simulink model "mqam_2020a"  (R2020a)
settings: Solver=VariableStepAuto  StartTime=0.0  StopTime=10.0  RelTol=1e-3
PreLoadFcn:
  | %%% model parameters %%%
  | 
  | Rb = 10e6; % bit rate
  | Tb = 1/Rb; % bit interval
  | 
  | M = 256; % constelation alphabet
  | Nb = log2(M); % number of bit
  | 
  | Rs = Rb/Nb; % symbol rate
  | N = 100; % number of samples per symbol
  | R = N*Rs; % sampling rate
  | 
  | fc = 100e6; % carrier frequency
  | 
  | Eg = 1 %
  | 
  | 
  | %%% gray code mapper %%%
  | 
  | gray_codes = get_gray_codes(Nb/2);
  | 
  | gray_cont = containers.Map % container
  | for i=1:size(gray_codes,2)
  |   binary_str = num2str(flip(gray_codes(:,i)'));
  |   binary_str(binary_str == ' ') = '';
  |   gray_cont(binary_str) = (i-1)*2 - ((M/4 -1)*2 + 1);
  | end
InitFcn:
  | phi = 0; % phase offset
undefined symbols (not defined in the file or in its folder): fdesignblkfcn, gcbh, magnitude
libraries: dspstat3 x3, dspsrcs4 x3, commchan3 x1, commfilt2 x1, commrandsrc3 x1, dsparch4 x1, commsink2 x1
settings Model: Creator=tapyu  LastModifiedBy=tapyu
settings DebuggingCC: UnconnectedInputMsg=none  UnconnectedOutputMsg=none  UnconnectedLineMsg=none  SFMachineParentedDataDiag=error

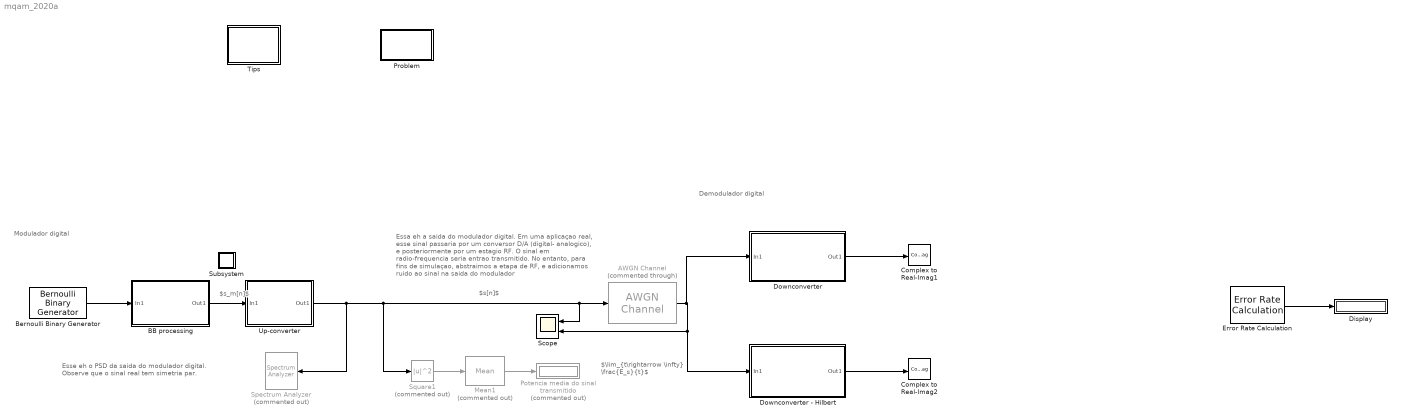
== system mqam_2020a ==
  note: Demodulador digital
  note: Essa eh a saida do modulador digital. Em uma aplicaçao
      | real, esse sinal passaria por um conversor D/A (digital-
      | analogico), e posteriormente por um estagio RF. O sinal
      | em radio-frequencia seria entrao transmitido. No entanto,
      | para fins de simulaçao, abstraimos a etapa de RF,
      | e adicionamos ruido ao sinal na saida do modulador
  note: $s[n]$
  note: Esse eh o PSD da saida do modulador digital.
      | Observe que o sinal real tem simetria par.
  note: Modulador digital
  note: $s_m[n]$
  note: $\lim_{t\rightarrow \infty} \frac{E_s}{t}$
  AWGN Channel : commchan3/AWGN Channel  Commented=through  InputProcessing=Columns as channels (frame based)  seed=67  noiseMode="Signal to noise ratio  (Eb/No)"  EbNodB=10  EsNodB=10  SNRdB=10  bitsPerSym=sqrt(M)  Ps=1  Tsym=Tb  variance=1
  BB processing : Subsystem
  Bernoulli Binary Generator : commrandsrc3/Bernoulli Binary Generator  ProbabilityOfZero=0.5  SeedSource=Auto  Seed=0  SampleTime=Tb  SamplesPerFrame=1  OutputDataType=double  SimulateUsing=Interpreted execution
  Complex to Real-Imag1 : ComplexToRealImag
  Complex to Real-Imag2 : ComplexToRealImag
  Display : Display
  Downconverter : Subsystem
  Downconverter - Hilbert : Subsystem
  Error Rate Calculation : commsink2/Error Rate Calculation  N=0  st_delay=0  cp_mode=Entire frame  subframe=[]  PMode=Port  WsName=ErrorVec  RsMode2=off  stop=off  numErr=100  maxBits=1e6
  Mean1 : dspstat3/Mean  Commented=on  run=on  reset_popup=None  directionMode=Entire input  dimension=1  roiEnable=off  roiType=Rectangles  roiPortion=Entire ROI  roiOutput=Individual statistics for each ROI  roiFlag=off  roundingMode=Floor  overflowMode=off  outputDataTypeStr=Inherit: Same as accumulator  outputMin=[]  outputMax=[]  outputLastDataTypeStr=Inherit: Same as accumulator
  Potencia media do sinal transmitido : Display  Commented=on
  Problem : Subsystem
  Scope : Scope  NumInputPorts=2
  Spectrum Analyzer : SpectrumAnalyzer  Commented=on
  Square1 : Math  Commented=on  Operator=magnitude^2  SaturateOnIntegerOverflow=on
  Subsystem : Subsystem
  Tips : Subsystem
  Up-converter : Subsystem
  wires:
  BB processing/1(Out1) -> Up-converter/1(In1)
  Up-converter/1(Out1) -> Spectrum Analyzer/1, Square1/1, Scope/1, AWGN Channel/1
  Mean1/1 -> Potencia media do sinal transmitido/1
  Square1/1 -> Mean1/1
  AWGN Channel/1 -> Downconverter/1(In1), Downconverter - Hilbert/1(In1), Scope/2
  Bernoulli Binary Generator/1 -> BB processing/1(In1)
  Error Rate Calculation/1 -> Display/1
  Downconverter/1(Out1) -> Complex to Real-Imag1/1
  Downconverter - Hilbert/1(Out1) -> Complex to Real-Imag2/1

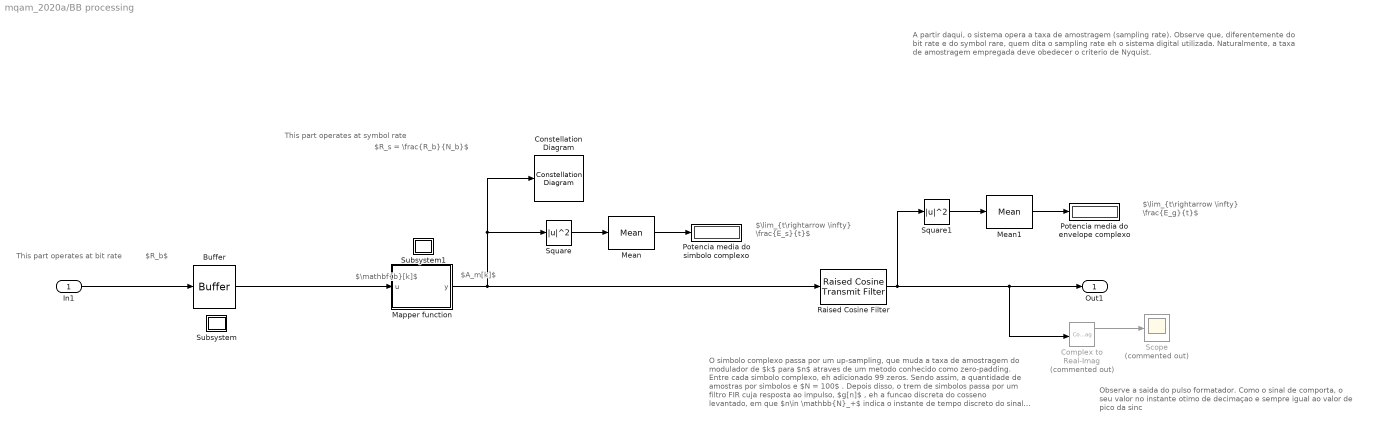
== system mqam_2020a/BB processing ==
  note: A partir daqui, o sistema opera a taxa de amostragem (sampling rate).
      | Observe que, diferentemente do bit rate e do symbol rare, quem dita o sampling rate
      | eh o sistema digital utilizada. Naturalmente, a taxa de amostragem empregada deve
      | obedecer o criterio de Nyquist.
  note: Observe a saida do pulso formatador. Como o sinal de comporta,
      | o seu valor no instante otimo de decimaçao e sempre igual ao
      | valor de pico da sinc
  note: $\lim_{t\rightarrow \infty} \frac{E_s}{t}$
  note: $R_s = \frac{R_b}{N_b}$
  note: This part operates
      | at symbol rate
  note: $R_b$
  note: This part operates at bit rate
  note: O simbolo complexo passa por um up-sampling, que muda a taxa de amostragem do modulador de $k$ para $n$ atraves de um metodo conhecido como zero-padding. Entre cada simbolo complexo, eh adicionado 99 zeros. Sendo assim, a quantidade de amostras por simbolos e $N = 100$ . Depois disso, o trem de simbolos passa por um filtro FIR cuja resposta ao impulso, $g[n]$ , eh a funcao discreta do cosseno levantado, em que $n\in \mathbb{N}_+$ indica o instante de tempo discreto do sinal que opera a taxa de amostragem, $R=N R_s$ . O sinal de saida do filtro para o k-esimo simbolo transmitido eh dado por $s[n] = A_m[k] g[n]$ . Este sinal eh comumente referido como envelope complexo. Clique no bloco do filtro cosseno levantado->view filter response e observe os seguintes pontos:
      |
      | - Resposta ao impulso do filtro cosseno levantado eh na verdade uma versao truncada da mesma em 4 intervalos de simbolos (recorde que cada intervalo de simbolos contem $N = 100$ amostras). O motivo disso eh a factibilidade na hora da implementaçao: nao eh possivel definir um filtro FIR com resposta ao impulso de duraçao infinita, por isso faz-se necessario trunca-la. Observe que o efeito to truncamento no tempo leva a uma distorçao da resposta em frequencia do filtro FIR. Tem-se entao um termo de compromisso (trade-off) entre o tramanho da janela de truncamento e nivel de distorçao da resposta de frequencia.
      |
      | - Oberseve que, embora haja sobreposiçao entre os simbolos vizinhos, ha interferencia nula nos instantes otimos de decimaçao: conte $100$ amostras a partir do instante de pico e vera que pulso cruza o valor zero nesses instantes. Isso ocorre porque o pulso cosseno levantado respeita o criterio de Nyquist de nao ISI.
      |
      | - A amplitude do cosseno levantado eh modificada de tal forma que $E_g = 1$$
  note: $A_m[k]$
  note: $\mathbf{b}[k]$
  note: $\lim_{t\rightarrow \infty} \frac{E_g}{t}$
  In1 : Inport
  Buffer : Buffer  N=Nb  OutputFrames=off
  Complex to Real-Imag : ComplexToRealImag  Commented=on
  Constellation Diagram : ConstellationDiagram
  Mapper function : MATLAB Function  TreatAsAtomicUnit=on
  Mean : dspstat3/Mean  run=on  reset_popup=None  directionMode=Entire input  dimension=1  roiEnable=off  roiType=Rectangles  roiPortion=Entire ROI  roiOutput=Individual statistics for each ROI  roiFlag=off  roundingMode=Floor  overflowMode=off  outputDataTypeStr=Inherit: Same as accumulator  outputMin=[]  outputMax=[]  outputLastDataTypeStr=Inherit: Same as accumulator
  Mean1 : dspstat3/Mean  run=on  reset_popup=None  directionMode=Entire input  dimension=1  roiEnable=off  roiType=Rectangles  roiPortion=Entire ROI  roiOutput=Individual statistics for each ROI  roiFlag=off  roundingMode=Floor  overflowMode=off  outputDataTypeStr=Inherit: Same as accumulator  outputMin=[]  outputMax=[]  outputLastDataTypeStr=Inherit: Same as accumulator
  Potencia media do envelope complexo : Display
  Potencia media do simbolo complexo : Display
  Raised Cosine Filter : commfilt2/Raised Cosine Transmit Filter  filtType=Normal  R=0.2  filtSpan=4  N=N  filterGain=sqrt(N)  RateOptions=Allow multirate processing  framing=Mute  checkCoeff=off  variableName=rcTxFilt  checkGain=Normalized  sampMode=Mute  saveAsFlag=0  currentFiltSpan=4  D=(4)/2  launchFVT=on  roundingMode=Floor  overflowMode=off  coeffDataTypeStr=Inherit: Same word length as input  coeffMin=[]  coeffMax=[]  coeffLastDataTypeStr=Inherit: Same word length as input  outputDataTypeStr=Inherit: Same as accumulator  outputMin=[]  outputMax=[]  outputLastDataTypeStr=Inherit: Same as accumulator
  Scope : Scope  Commented=on
  Square : Math  Operator=magnitude^2  SaturateOnIntegerOverflow=on
  Square1 : Math  Operator=magnitude^2  SaturateOnIntegerOverflow=on
  Subsystem : Subsystem
  Subsystem1 : Subsystem
  Out1 : Outport
  wires:
  Buffer/1 -> Mapper function/1(u)
  Mean/1 -> Potencia media do simbolo complexo/1
  Mapper function/1(y) -> Constellation Diagram/1, Square/1, Raised Cosine Filter/1
  Square/1 -> Mean/1
  In1/1 -> Buffer/1
  Mean1/1 -> Potencia media do envelope complexo/1
  Square1/1 -> Mean1/1
  Complex to Real-Imag/1 -> Scope/1
  Raised Cosine Filter/1 -> Complex to Real-Imag/1, Out1/1, Square1/1

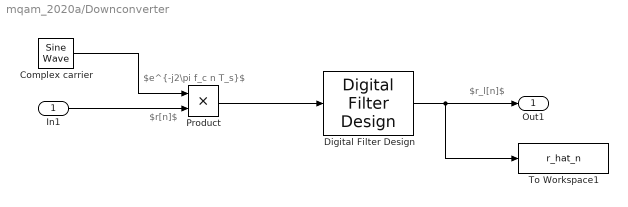
== system mqam_2020a/Downconverter ==
  note: $r[n]$
  note: $e^{-j2\pi f_c n T_s}$
  note: $r_l[n]$
  In1 : Inport
  Complex carrier : dspsrcs4/Sine Wave  Amplitude=sqrt(2/Eg)  Frequency=fc  Phase=0  SampleMode=Discrete  OutComplex=Complex  CompMethod=Trigonometric fcn  TableSize=Speed  SampleTime=1/R  SamplesPerFrame=1  ResetState=Restart at time zero  OutputFrames=off  dataType=double  wordLen=16  udDataType=sfix(16)  fracBitsMode=Best precision  numFracBits=15  OutDataTypeStr=double  LastOutDataTypeStr=double
  Digital Filter Design : dsparch4/Digital Filter Design  mwdsp_browser_bugfix_var=off
  Product : Product
  To Workspace1 : ToWorkspace  VariableName=r_hat_n  SaveFormat=Timeseries  SampleTime=-1
  Out1 : Outport
  wires:
  In1/1 -> Product/2
  Complex carrier/1 -> Product/1
  Product/1 -> Digital Filter Design/1
  Digital Filter Design/1 -> To Workspace1/1, Out1/1

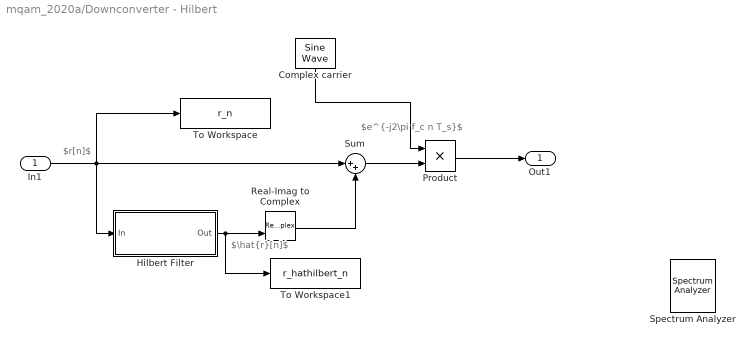
== system mqam_2020a/Downconverter - Hilbert ==
  note: $e^{-j2\pi f_c n T_s}$
  note: $r[n]$
  note: $\hat{r}[n]$
  In1 : Inport
  Complex carrier : dspsrcs4/Sine Wave  Amplitude=sqrt(2/Eg)  Frequency=-fc  Phase=0  SampleMode=Discrete  OutComplex=Complex  CompMethod=Trigonometric fcn  TableSize=Speed  SampleTime=1/R  SamplesPerFrame=1  ResetState=Restart at time zero  OutputFrames=off  dataType=double  wordLen=16  udDataType=sfix(16)  fracBitsMode=Best precision  numFracBits=15  OutDataTypeStr=double  LastOutDataTypeStr=double
  Hilbert Filter : Subsystem  DialogController=fdesignblkfcn  InitFcn=fdesignblkfcn(gcbh, {'InitFcn'});  mask(Hilbert Filter){}
      mask help: Design a Hilbert filter
      settings: CopyFcn=fdesignblkfcn(gcbh, {'CopyFcn'});
      mask Help: helpview(mapfilelocation('dsp'), 'dsphilbertfilter');
      mask Display: disp('Hilbert')
  Product : Product
  Real-Imag to Complex : RealImagToComplex
  Spectrum Analyzer : SpectrumAnalyzer  NumInputPorts=2
  Sum : Sum  Inputs=|++
  To Workspace : ToWorkspace  VariableName=r_n  SaveFormat=Timeseries  SampleTime=-1
  To Workspace1 : ToWorkspace  VariableName=r_hathilbert_n  SaveFormat=Timeseries  SampleTime=-1
  Out1 : Outport
  wires:
  Sum/1 -> Product/2
  Complex carrier/1 -> Product/1
  Product/1 -> Out1/1
  In1/1 -> Sum/1, To Workspace/1, Hilbert Filter/1(In)
  Hilbert Filter/1(Out) -> To Workspace1/1, Real-Imag to Complex/2
  Real-Imag to Complex/1 -> Sum/2

== system mqam_2020a/Problem ==
  note: Bit rate:

== system mqam_2020a/Subsystem ==
  note: This is the complex envelope, also called the low-pass equivalent of the modulation scheme.

== system mqam_2020a/Tips ==
  note: Tips:
      |
      | - Go to debug->information overlays to set/unset visual indicators (called overlays). The main ones are: colors, timing legend, signals dimensions, base data types
      | - Go to modeling->model explorer->mqam->callbacks->PreLoadFnc to see the variables declared in this Simulink model. They are visible in the workspace area of the main window. In addition they can also be changed in the command window.

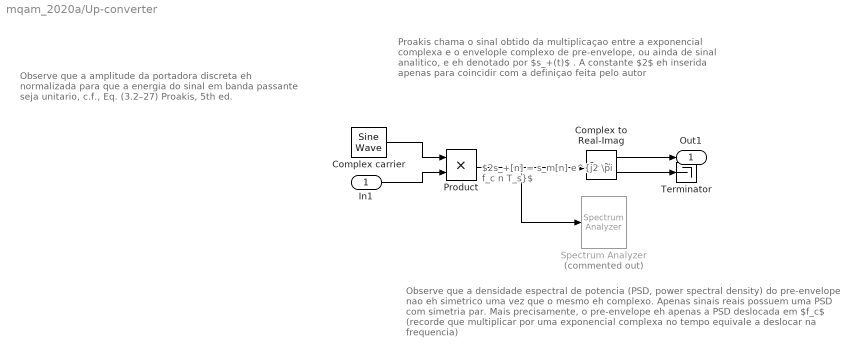
== system mqam_2020a/Up-converter ==
  note: Observe que a amplitude da portadora discreta eh
      | normalizada para que a energia do sinal em banda
      | passante seja unitario, c.f., Eq. (3.2–27) Proakis, 5th ed.
  note: Observe que a densidade espectral de potencia (PSD, power spectral density) do pre-envelope nao eh simetrico uma vez que o mesmo eh complexo.
      | Apenas sinais reais possuem uma PSD com simetria par. Mais precisamente, o pre-envelope eh apenas a PSD deslocada em $f_c$ (recorde que multiplicar por uma exponencial complexa no tempo equivale a deslocar na frequencia)
  note: Proakis chama o sinal obtido da multiplicaçao entre a exponencial
      | complexa e o envelople complexo de pre-envelope, ou ainda de
      | sinal analitico, e eh denotado por $s_+(t)$ . A constante $2$ eh inserida
      | apenas para coincidir com a definiçao feita pelo autor
  note: $2s_+[n] = s_m[n] e^{j2 \pi f_c n T_s}$
  In1 : Inport
  Complex carrier : dspsrcs4/Sine Wave  Amplitude=sqrt(2)  Frequency=fc  Phase=0  SampleMode=Discrete  OutComplex=Complex  CompMethod=Trigonometric fcn  TableSize=Speed  SampleTime=1/R  SamplesPerFrame=1  ResetState=Restart at time zero  OutputFrames=off  dataType=double  wordLen=16  udDataType=sfix(16)  fracBitsMode=Best precision  numFracBits=15  OutDataTypeStr=double  LastOutDataTypeStr=double
  Complex to Real-Imag : ComplexToRealImag
  Product : Product
  Spectrum Analyzer : SpectrumAnalyzer  Commented=on
  Terminator : Terminator
  Out1 : Outport
  wires:
  Complex carrier/1 -> Product/1
  In1/1 -> Product/2
  Complex to Real-Imag/1 -> Out1/1
  Product/1 -> Spectrum Analyzer/1, Complex to Real-Imag/1
  Complex to Real-Imag/2 -> Terminator/1

== system mqam_2020a/BB processing/Subsystem ==
  note: The bitstream operates at a rate of $R_b = 10 Mbps$ . The first task is to transform the stream bit into a vector, $\mathbf{b}[k] \in \mathbb{R}^{K}$ , where $k \in \mathbb{N}_+$ is the $k$ th set of $K = \log_2 (M)$ bits

== system mqam_2020a/BB processing/Subsystem1 ==
  note: Each sequence of $K = \log_2(M)$ bit is mapped (using Gray code) to a complex symbol, $A_m[k]$ , where $m \in \{1,2,\cdots,M\}$ is the $m$ th complex symbol of the alphabet, and $k \in \mathbb{N}_+$ is the $k$ th transmitted symbol

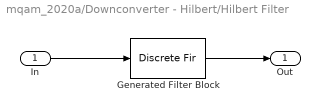
== system mqam_2020a/Downconverter - Hilbert/Hilbert Filter ==
  In : Inport
  Generated Filter Block : DiscreteFir  Tag=BlockMethodSubSystem  Coefficients=[-0.379139248397066475 -6.14990643046237073e-15 -0.0322139499300219123 -1.08779359218186267e-15 -0.0337279953162739066 -1.6870185803874449e-15 -0.0362439670869629804 -2.70443389904784226e-15 -0.0398003827467814375 5.01855501600090292e-15 -0.0445494339270779971 -2.66236685475540469e-15 -0.0508633445439188314 5.47305256670682638e-16 -0.0595171048736182762 -1.85441939581920678e-15 -0.0720795865005312564 7.71951946809679157e-16 -0.0919627441700265891 -6.38378239159465011e-16 -0.128017407479324774 1.11022302462515654e-16 -0.212602811441472639 -3.26128013483639734e-16 -0.636747756767987561 0 0.636747756767987561 3.26128013483639734e-16 0.212602811441472639 -1.11022302462515654e-16 0.128017407479324774 6.38378239159465011e-16 0.0919627441700265891 -7.71951946809679157e-16 0.0720795865005312564 1.85441939581920678e-15 0.0595171048736182762 -5.47305256670682638e-16 0.0508633445439188314 2.66236685475540469e-15 0.0445494339270779971 -5.01855501600090292e-15 0.0398003827467814375 2.70443389904784226e-15 0.0362439670869629804 1.6870185803874449e-15 0.0337279953162739066 1.08779359218186267e-15 0.0322139499300219123 6.14990643046237073e-15 0.379139248397066475]
  Out : Outport  VectorParamsAs1DForOutWhenUnconnected=off
  wires:
  Generated Filter Block/1 -> Out/1
  In/1 -> Generated Filter Block/1

== matlab function mqam_2020a/BB processing/Mapper function ==
  data: u input; y output; gray_codes parameter; M parameter
function y = fcn(u, gray_codes, M)

v = [u(1:end/2), u(end/2+1:end)];
w = zeros(2,1);

for i = 1:2
    for j = 1:size(gray_codes,2)
        if all(gray_codes(:,j) == v(:,i))
            w(i) = (j-1)*2 - (sqrt(M) - 1);
            break
        end
    end
end

y = w(1) + 1j*w(2);
end
